simulink model "svpwm_test"  (R2026a)
settings: Solver=VariableStepAuto  StopTime=0.006
libraries: mcbeeMathTransformLib x2, simulink x1, eePwmGeneratorTwoLevel x1

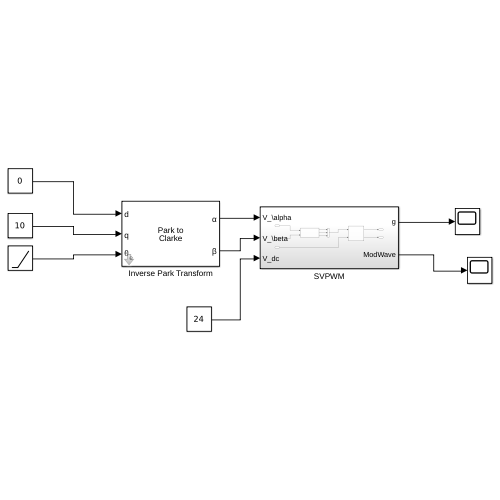
[thumbnail: Simulink's stored preview of the top-level diagram]
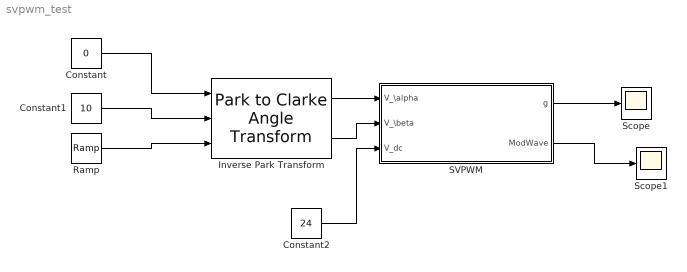
== system svpwm_test ==
  Constant : Constant  Value=0
  Constant1 : Constant  Value=10
  Constant2 : Constant  Value=24
  Inverse Park Transform : mcbeeMathTransformLib/Park to Clarke Angle Transform  AxisAlignment=D-axis  UseWithEmbedded=on  PhaseInput=Two inputs  ThetaInput=Electrical position  AngleInput=Radians  N_points=1024
      settings: LibrarySourceBlock=mcbhdllib/Controls/Math Transforms/Inverse Park Transform
  Ramp : simulink/Sources/Ramp  slope=pi/2/0.01  start=0  InitialOutput=0
  SVPWM : Subsystem
  Scope : Scope
      settings: ActiveDisplayYMinimum=-0.25817363083270917  ActiveDisplayYMaximum=1.2465176768418447
  Scope1 : Scope
      settings: ActiveDisplayYMinimum=-0.90210979560879023  ActiveDisplayYMaximum=0.90210979560879023
  wires:
  Inverse Park Transform/1 -> SVPWM/1(V_\alpha)
  Inverse Park Transform/2 -> SVPWM/2(V_\beta)
  Constant/1 -> Inverse Park Transform/1
  Constant1/1 -> Inverse Park Transform/2
  Ramp/1 -> Inverse Park Transform/3
  SVPWM/1(g) -> Scope/1
  SVPWM/2(ModWave) -> Scope1/1
  Constant2/1 -> SVPWM/3(V_dc)

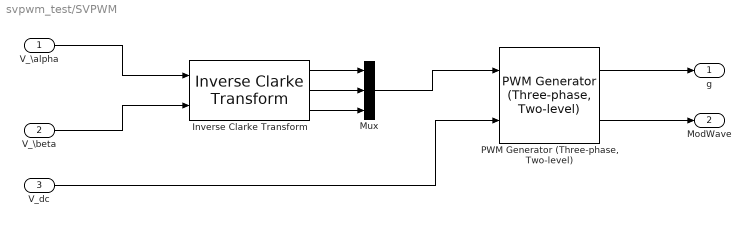
== system svpwm_test/SVPWM ==
  V_\alpha : Inport
  V_\beta : Inport  Port=2
  V_dc : Inport  Port=3
  Inverse Clarke Transform : mcbeeMathTransformLib/Inverse Clarke Transform  PowerInvariant=off  UseWithEmbedded=on  PhaseInput=Two inputs
      settings: LibrarySourceBlock=mcbhdllib/Controls/Math Transforms/Inverse Clarke Transform
  Mux : Mux  Inputs=3
  "PWM Generator (Three-phase, Two-level)" : eePwmGeneratorTwoLevel/PWM Generator (Three-phase, Two-level)  PWMMode=Continuous PWM (CPWM)  CPWMMode=SVM: space vector modulation  DPWMMode=60 DPWM: 60 degree discontinuous PWM  fsw=1e3  Ts=5e-5
      settings: LibrarySourceBlock=|
      | ee_sl_lib/Pulse Width
      | Modulation/PWM Generator
      | (Three-phase, Two-level)
  g : Outport
  ModWave : Outport  Port=2
  wires:
  V_\alpha/1 -> Inverse Clarke Transform/1
  V_\beta/1 -> Inverse Clarke Transform/2
  Inverse Clarke Transform/1 -> Mux/1
  Inverse Clarke Transform/2 -> Mux/2
  Inverse Clarke Transform/3 -> Mux/3
  Mux/1 -> "PWM Generator (Three-phase, Two-level)"/1
  "PWM Generator (Three-phase, Two-level)"/1 -> g/1
  "PWM Generator (Three-phase, Two-level)"/2 -> ModWave/1
  V_dc/1 -> "PWM Generator (Three-phase, Two-level)"/2
